simulink model "robot_circular"  (Simulink 8.2)
settings: Solver=FixedStepDiscrete  StartTime=0.0  StopTime=100  FixedStep=0.1  RelTol=1e-3
values from neighbouring files (symbols this model uses):
  Link1 = [pi/2, 0, pi/2, 0]    [robot_parameters.m]
  Link2 = [0, 0.404, pi/2, 0]    [robot_parameters.m]
  Link3 = [-pi/2, 0, 0, 0]    [robot_parameters.m]
  Link4 = [pi/2, 0.025, 0, 0.405]    [robot_parameters.m]
  Link5 = [pi/2, 0, pi/2, 0]    [robot_parameters.m]
  Link6 = [0, 0, pi/2, 0]    [robot_parameters.m]
  NoOfLinks = 6    [robot_parameters.m]
libraries: vrlib x3, instrumentlib x2, dspnetwork x2, simulink x2, utility x1
settings Model: Creator=angelosanto  LastModifiedBy=shashank  BufferReuse=off
settings DataIOCC: ReturnWorkspaceOutputs=on
settings OptimizationCC: BlockReduction=off  BooleanDataType=off  ConditionallyExecuteInputs=off  InlineParams=on  OptimizeBlockIOStorage=off  BufferReuse=off  ExpressionFolding=off  LocalBlockOutputs=off
settings RTWCC: GenCodeOnly=on  GenerateMakefile=off

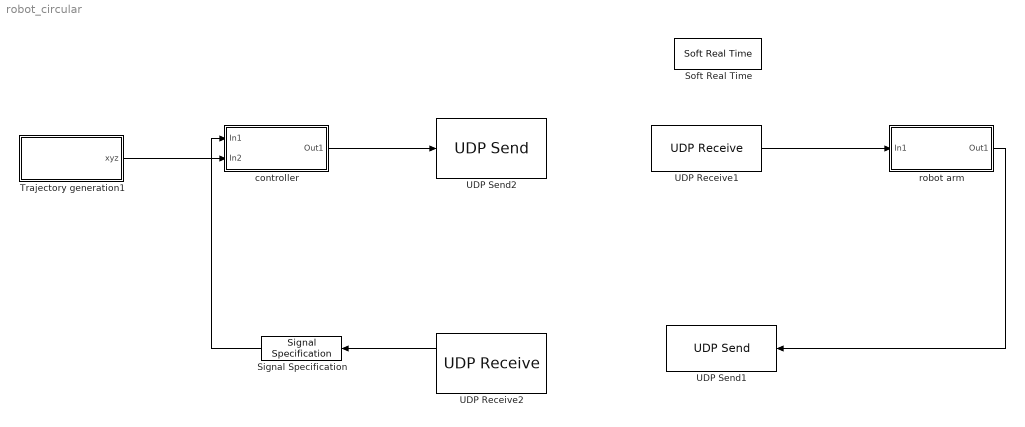
== system robot_circular ==
  Signal Specification : SignalSpecification  OutMin=6  OutMax=6  OutDataTypeStr=double
      settings: LockScale=on
  Soft Real Time : utility/Soft Real Time  x=0.5
  Trajectory generation1 : Subsystem
  UDP Receive1 : instrumentlib/UDP Receive  Priority=3  Host=localhost  Port=9090  LocalPort=9090  DataSize="[6  1]"  EnableBlockingMode=on  Timeout=10  SampleTime=0.1  DataType=double  ByteOrder=BigEndian
  UDP Receive2 : dspnetwork/UDP Receive  localURL='0.0.0.0'  localPort=9093  remoteURL='0.0.0.0'  remotePort=-1  recvBufferSize=8192  dims=6  signalDatatype=double  isVarSize=off  showBlockingTime=on  blockingTime=inf  sampletime=0.1  blockPlatform=LINUX
  UDP Send1 : instrumentlib/UDP Send  Priority=5  Host=localhost  Port=9092  LocalPort=9092  EnableBlockingMode=on  ByteOrder=BigEndian
  UDP Send2 : dspnetwork/UDP Send  remoteURL='localhost'  remotePort=9090  localURL='0.0.0.0'  localPortSource=Specify via dialog  localPort=9091  sampletime=-1  blockPlatform=LINUX  separateLengthPort=0
  controller : Subsystem
  robot arm : Subsystem  Priority=4
  wires:
  UDP Receive1/1 -> robot arm/1(In1)
  robot arm/1(Out1) -> UDP Send1/1
  controller/1(Out1) -> UDP Send2/1
  Trajectory generation1/1(xyz) -> controller/2(In2)
  UDP Receive2/1 -> Signal Specification/1
  Signal Specification/1 -> controller/1(In1)

== system robot_circular/Trajectory generation1 ==
  Bus Creator : BusCreator  Inputs='x','y','z'
  Constant1 : Constant  Value=0
  Constant4 : Constant
  Display : Display
  Fcn : Fcn  Expr=0.1*cos(u)+0.5
  Fcn1 : Fcn  Expr=0.1*sin(u)
  Fcn2 : Fcn  Expr=u/30
  Memory1 : Memory
  Sum1 : Sum  Inputs=|++
  xyz : Outport
  wires:
  Constant4/1 -> Sum1/2
  Sum1/1 -> Memory1/1, Display/1, Fcn2/1
  Memory1/1 -> Sum1/1
  Bus Creator/1 -> xyz/1
  Fcn1/1 -> Bus Creator/2  "y"
  Fcn/1 -> Bus Creator/1  "x"
  Fcn2/1 -> Fcn1/1, Fcn/1
  Constant1/1 -> Bus Creator/3  "z"

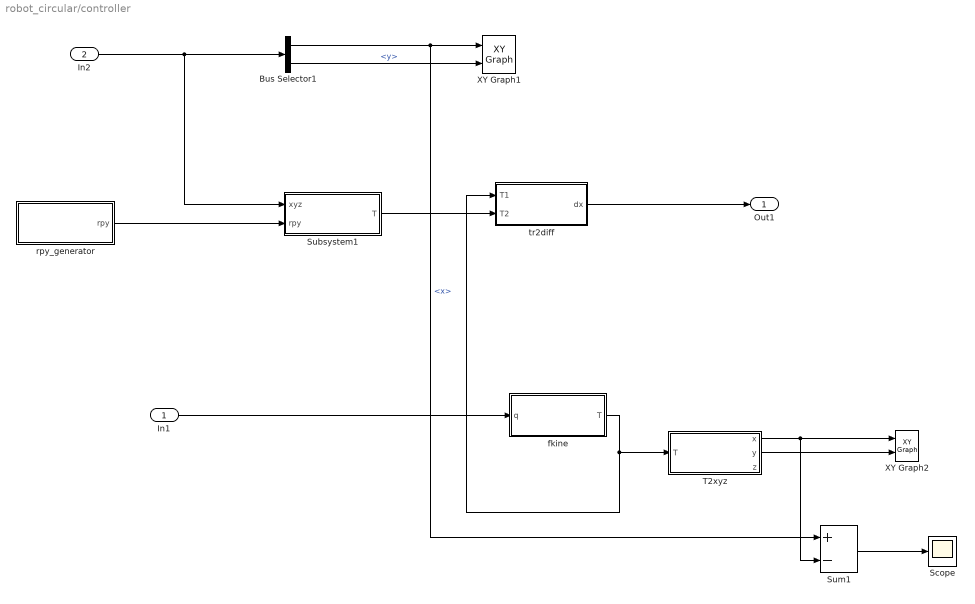
== system robot_circular/controller ==
  In1 : Inport
  In2 : Inport  Port=2
  Bus Selector1 : BusSelector  OutputSignals=x,y
  Scope : Scope
      settings: YMin=-0.03  YMax=-0.01
  Subsystem1 : Subsystem
  Sum1 : Sum  Inputs=+-
  T2xyz : Subsystem
  XY Graph1 : simulink/Sinks/XY Graph  xmin=-0.2  xmax=0.8  ymin=-0.5  ymax=0.5  st=-1
  XY Graph2 : simulink/Sinks/XY Graph  xmin=-0.2  xmax=0.8  ymin=-0.5  ymax=0.5  st=-1
  fkine : Subsystem  TreatAsAtomicUnit=on
  rpy_generator : Subsystem
  tr2diff : Subsystem
  Out1 : Outport
  wires:
  T2xyz/1(x) -> Sum1/2, XY Graph2/1
  fkine/1(T) -> tr2diff/1(T1), T2xyz/1(T)
  rpy_generator/1(rpy) -> Subsystem1/2(rpy)
  Bus Selector1/1 -> Sum1/1, XY Graph1/1  "<x>"
  Subsystem1/1(T) -> tr2diff/2(T2)
  Sum1/1 -> Scope/1
  Bus Selector1/2 -> XY Graph1/2  "<y>"
  T2xyz/2(y) -> XY Graph2/2
  In2/1 -> Subsystem1/1(xyz), Bus Selector1/1
  tr2diff/1(dx) -> Out1/1
  In1/1 -> fkine/1(q)

== system robot_circular/robot arm ==
  In1 : Inport
  Delay : Memory  X0=[pi/2; pi/2; 0; 0; pi/2; pi/2]  InheritSampleTime=on
  Gain1 : Gain  Gain=0.1
  Product : Product  Multiplication=Matrix(*)  RndMeth=Zero
  Scope5 : Scope
      settings: YMin=-0.02  YMax=0.0175  SaveName=ScopeData2
  Sum : Sum
  ijacob : Product  Inputs=/  Multiplication=Matrix(*)  RndMeth=Zero
  jacobn : Subsystem  TreatAsAtomicUnit=on
  Out1 : Outport
  wires:
  jacobn/1(Out1) -> ijacob/1
  ijacob/1 -> Product/1
  Sum/1 -> Delay/1
  Delay/1 -> Out1/1, jacobn/1(q), Sum/2
  Product/1 -> Gain1/1
  Gain1/1 -> Scope5/1, Sum/1
  In1/1 -> Product/2

== system robot_circular/controller/Subsystem1 ==
  xyz : Inport
  rpy : Inport  Port=2
  Bus Selector : BusSelector  OutputSignals=x,y,z
  Bus Selector1 : BusSelector  OutputSignals=roll,pitch,yaw
  Product : Product  Multiplication=Matrix(*)  RndMeth=Zero
  rpy2T : Subsystem
  xyz2T : Subsystem
  T : Outport
  wires:
  xyz/1 -> Bus Selector/1
  Bus Selector/1 -> xyz2T/1(x)  "<x>"
  Bus Selector/2 -> xyz2T/2(y)  "<y>"
  Bus Selector/3 -> xyz2T/3(z)  "<z>"
  xyz2T/1(T) -> Product/1
  Product/1 -> T/1
  rpy2T/1(T) -> Product/2
  rpy/1 -> Bus Selector1/1
  Bus Selector1/1 -> rpy2T/1(roll)  "<roll>"
  Bus Selector1/2 -> rpy2T/2(pitch)  "<pitch>"
  Bus Selector1/3 -> rpy2T/3(yaw)  "<yaw>"

== system robot_circular/controller/T2xyz ==
  T : Inport
  Selector : Selector  NumberOfDimensions=2  InputPortWidth=3  IndexOptions=Index vector (dialog),Index vector (dialog)  Indices=1,4  OutputSizes=1,1
  Selector1 : Selector  NumberOfDimensions=2  InputPortWidth=3  IndexOptions=Index vector (dialog),Index vector (dialog)  Indices=2,4  OutputSizes=1,1
  Selector2 : Selector  NumberOfDimensions=2  InputPortWidth=3  IndexOptions=Index vector (dialog),Index vector (dialog)  Indices=3,4  OutputSizes=1,1
  x : Outport
  y : Outport  Port=2
  z : Outport  Port=3
  wires:
  Selector/1 -> x/1
  Selector1/1 -> y/1
  Selector2/1 -> z/1
  T/1 -> Selector/1, Selector2/1, Selector1/1

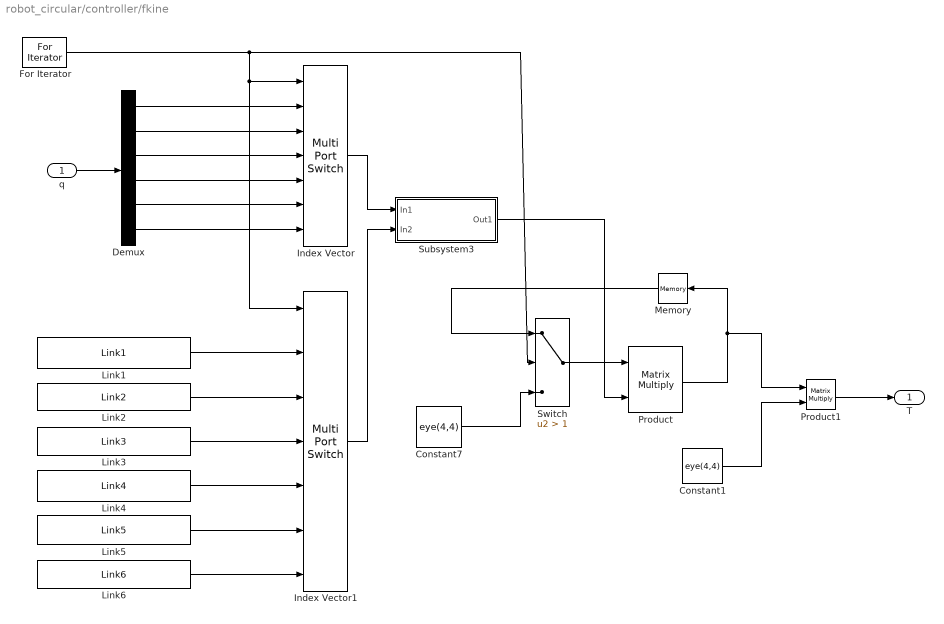
== system robot_circular/controller/fkine ==
  q : Inport
  Constant1 : Constant  Value=eye(4,4)
  Constant7 : Constant  Value=eye(4,4)
  Demux : Demux  Outputs=6
  For Iterator : ForIterator  IterationLimit=NoOfLinks
  Index Vector : MultiPortSwitch  Inputs=6
  Index Vector1 : MultiPortSwitch  Inputs=6
  Link1 : Constant  Value=Link1
  Link2 : Constant  Value=Link2
  Link3 : Constant  Value=Link3
  Link4 : Constant  Value=Link4
  Link5 : Constant  Value=Link5
  Link6 : Constant  Value=Link6
  Memory : Memory  X0=eye(4,4)  InheritSampleTime=on
  Product : Product  Multiplication=Matrix(*)  RndMeth=Zero
  Product1 : Product  Multiplication=Matrix(*)  RndMeth=Zero
  Subsystem3 : Subsystem
  Switch : Switch  Criteria=u2 > Threshold  Threshold=1
  T : Outport
  wires:
  Memory/1 -> Switch/1
  Switch/1 -> Product/1
  Subsystem3/1(Out1) -> Product/2
  Constant7/1 -> Switch/3
  Product/1 -> Product1/1, Memory/1
  Index Vector1/1 -> Subsystem3/2(In2)
  Index Vector/1 -> Subsystem3/1(In1)
  Demux/6 -> Index Vector/7
  Demux/5 -> Index Vector/6
  Demux/4 -> Index Vector/5
  Demux/3 -> Index Vector/4
  Demux/2 -> Index Vector/3
  Demux/1 -> Index Vector/2
  q/1 -> Demux/1
  Link6/1 -> Index Vector1/7
  Link5/1 -> Index Vector1/6
  Link4/1 -> Index Vector1/5
  Link3/1 -> Index Vector1/4
  Link2/1 -> Index Vector1/3
  Link1/1 -> Index Vector1/2
  For Iterator/1 -> Switch/2, Index Vector1/1, Index Vector/1
  Product1/1 -> T/1
  Constant1/1 -> Product1/2

== system robot_circular/controller/rpy_generator ==
  Bus Creator1 : BusCreator  Inputs=3
  Constant : Constant  Value=0  VectorParams1D=off
  Constant2 : Constant  Value=0
  Constant3 : Constant  Value=0
  rpy : Outport
  wires:
  Constant2/1 -> Bus Creator1/2  "pitch"
  Constant/1 -> Bus Creator1/1  "roll"
  Constant3/1 -> Bus Creator1/3  "yaw"
  Bus Creator1/1 -> rpy/1

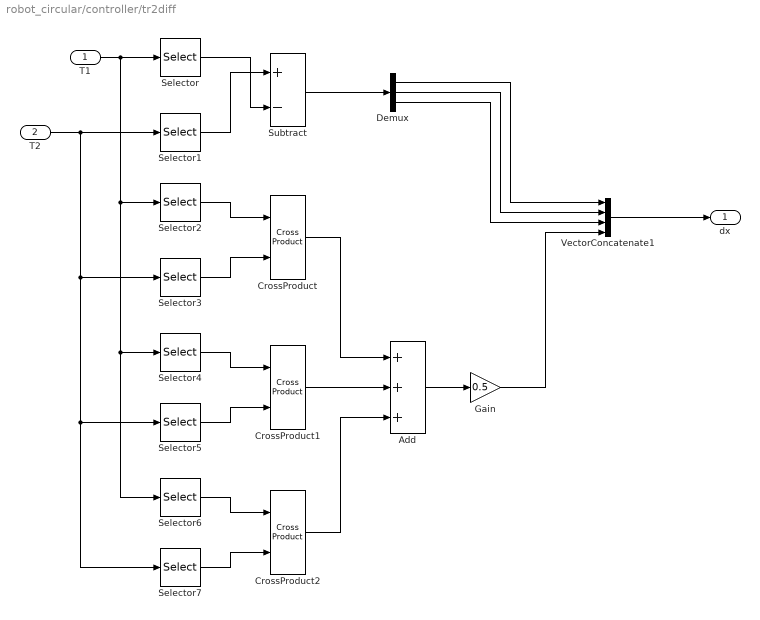
== system robot_circular/controller/tr2diff ==
  T1 : Inport
  T2 : Inport  Port=2
  Add : Sum  Inputs=+++
  CrossProduct : vrlib/Utilities/Cross Product
  CrossProduct1 : vrlib/Utilities/Cross Product
  CrossProduct2 : vrlib/Utilities/Cross Product
  Demux : Demux  Outputs=3
  Gain : Gain  Gain=0.5
  Selector : Selector  NumberOfDimensions=2  InputPortWidth=3  IndexOptions=Index vector (dialog),Index vector (dialog)  Indices=[1:3],4  OutputSizes=1,1
  Selector1 : Selector  NumberOfDimensions=2  InputPortWidth=3  IndexOptions=Index vector (dialog),Index vector (dialog)  Indices=[1:3],4  OutputSizes=1,1
  Selector2 : Selector  NumberOfDimensions=2  InputPortWidth=3  IndexOptions=Index vector (dialog),Index vector (dialog)  Indices=[1:3],1  OutputSizes=1,1
  Selector3 : Selector  NumberOfDimensions=2  InputPortWidth=3  IndexOptions=Index vector (dialog),Index vector (dialog)  Indices=[1:3],1  OutputSizes=1,1
  Selector4 : Selector  NumberOfDimensions=2  InputPortWidth=3  IndexOptions=Index vector (dialog),Index vector (dialog)  Indices=[1:3],2  OutputSizes=1,1
  Selector5 : Selector  NumberOfDimensions=2  InputPortWidth=3  IndexOptions=Index vector (dialog),Index vector (dialog)  Indices=[1:3],2  OutputSizes=1,1
  Selector6 : Selector  NumberOfDimensions=2  InputPortWidth=3  IndexOptions=Index vector (dialog),Index vector (dialog)  Indices=[1:3],3  OutputSizes=1,1
  Selector7 : Selector  NumberOfDimensions=2  InputPortWidth=3  IndexOptions=Index vector (dialog),Index vector (dialog)  Indices=[1:3],3  OutputSizes=1,1
  Subtract : Sum  Inputs=+-
  VectorConcatenate1 : Concatenate  NumInputs=4
  dx : Outport
  wires:
  T1/1 -> Selector/1, Selector2/1, Selector6/1, Selector4/1
  T2/1 -> Selector1/1, Selector7/1, Selector5/1, Selector3/1
  Selector1/1 -> Subtract/1
  Selector/1 -> Subtract/2
  Selector2/1 -> CrossProduct/1
  Selector3/1 -> CrossProduct/2
  Selector4/1 -> CrossProduct1/1
  Selector5/1 -> CrossProduct1/2
  Selector6/1 -> CrossProduct2/1
  Selector7/1 -> CrossProduct2/2
  CrossProduct/1 -> Add/1
  CrossProduct1/1 -> Add/2
  CrossProduct2/1 -> Add/3
  Add/1 -> Gain/1
  VectorConcatenate1/1 -> dx/1
  Subtract/1 -> Demux/1
  Demux/1 -> VectorConcatenate1/1
  Demux/2 -> VectorConcatenate1/2
  Demux/3 -> VectorConcatenate1/3
  Gain/1 -> VectorConcatenate1/4

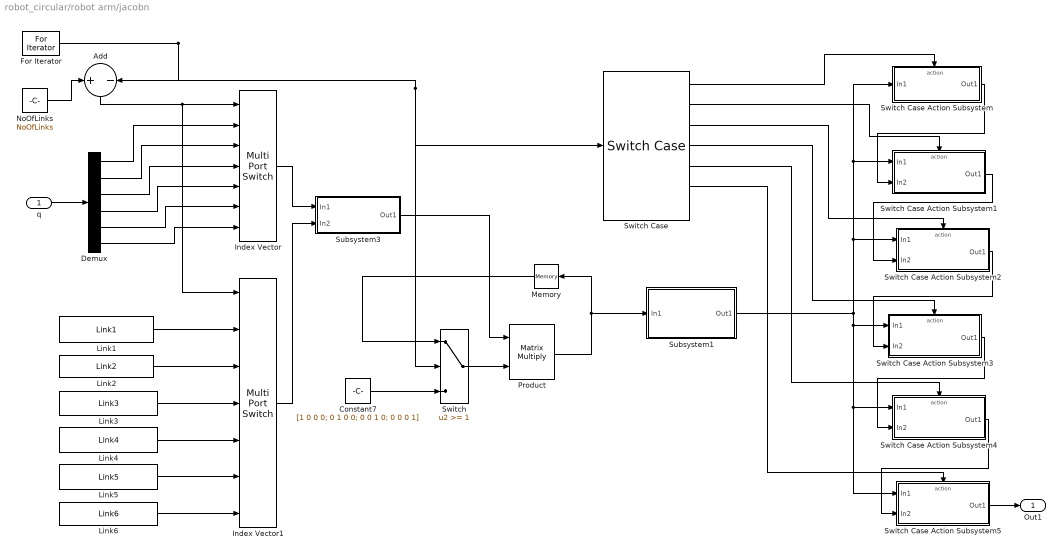
== system robot_circular/robot arm/jacobn ==
  q : Inport
  Add : Sum  Inputs=+-
  Constant7 : Constant  Value=[1 0 0 0; 0 1 0 0; 0 0 1 0; 0 0 0 1]
  Demux : Demux  Outputs=6
  For Iterator : ForIterator  IterationLimit=NoOfLinks
  Index Vector : MultiPortSwitch  DataPortOrder=Zero-based contiguous  Inputs=6  zeroidx=on
  Index Vector1 : MultiPortSwitch  DataPortOrder=Zero-based contiguous  Inputs=6  zeroidx=on
  Link1 : Constant  Value=Link1
  Link2 : Constant  Value=Link2
  Link3 : Constant  Value=Link3
  Link4 : Constant  Value=Link4
  Link5 : Constant  Value=Link5
  Link6 : Constant  Value=Link6
  Memory : Memory  X0=[1 0 0 0; 0 1 0 0; 0 0 1 0; 0 0 0 1]  InheritSampleTime=on
  NoOfLinks : Constant  Value=NoOfLinks
  Product : Product  Multiplication=Matrix(*)  RndMeth=Zero
  Subsystem1 : Subsystem
  Subsystem3 : Subsystem
  Switch : Switch  Threshold=1
  Switch Case : SwitchCase  CaseConditions={1, 2, 3, 4, 5, 6}
  Switch Case Action Subsystem : Subsystem  TreatAsAtomicUnit=on
  Switch Case Action Subsystem1 : Subsystem  TreatAsAtomicUnit=on
  Switch Case Action Subsystem2 : Subsystem  TreatAsAtomicUnit=on
  Switch Case Action Subsystem3 : Subsystem  TreatAsAtomicUnit=on
  Switch Case Action Subsystem4 : Subsystem  TreatAsAtomicUnit=on
  Switch Case Action Subsystem5 : Subsystem  TreatAsAtomicUnit=on
  Out1 : Outport
  wires:
  NoOfLinks/1 -> Add/1
  For Iterator/1 -> Add/2, Switch/2, Switch Case/1
  Add/1 -> Index Vector/1, Index Vector1/1
  Link1/1 -> Index Vector1/2
  Link2/1 -> Index Vector1/3
  Link3/1 -> Index Vector1/4
  Link4/1 -> Index Vector1/5
  Link5/1 -> Index Vector1/6
  Link6/1 -> Index Vector1/7
  q/1 -> Demux/1
  Demux/1 -> Index Vector/2
  Demux/2 -> Index Vector/3
  Demux/3 -> Index Vector/4
  Demux/4 -> Index Vector/5
  Demux/5 -> Index Vector/6
  Demux/6 -> Index Vector/7
  Index Vector/1 -> Subsystem3/1(In1)
  Index Vector1/1 -> Subsystem3/2(In2)
  Product/1 -> Memory/1, Subsystem1/1(In1)
  Constant7/1 -> Switch/3
  Subsystem3/1(Out1) -> Product/1
  Switch/1 -> Product/2
  Memory/1 -> Switch/1
  Subsystem1/1(Out1) -> Switch Case Action Subsystem/1(In1), Switch Case Action Subsystem1/1(In1), Switch Case Action Subsystem2/1(In1), Switch Case Action Subsystem5/1(In1), Switch Case Action Subsystem4/1(In1), Switch Case Action Subsystem3/1(In1)
  Switch Case/1 -> Switch Case Action Subsystem/Action
  Switch Case/2 -> Switch Case Action Subsystem1/Action
  Switch Case/3 -> Switch Case Action Subsystem2/Action
  Switch Case/4 -> Switch Case Action Subsystem3/Action
  Switch Case/5 -> Switch Case Action Subsystem4/Action
  Switch Case/6 -> Switch Case Action Subsystem5/Action
  Switch Case Action Subsystem5/1(Out1) -> Out1/1
  Switch Case Action Subsystem1/1(Out1) -> Switch Case Action Subsystem2/2(In2)
  Switch Case Action Subsystem/1(Out1) -> Switch Case Action Subsystem1/2(In2)
  Switch Case Action Subsystem2/1(Out1) -> Switch Case Action Subsystem3/2(In2)
  Switch Case Action Subsystem3/1(Out1) -> Switch Case Action Subsystem4/2(In2)
  Switch Case Action Subsystem4/1(Out1) -> Switch Case Action Subsystem5/2(In2)

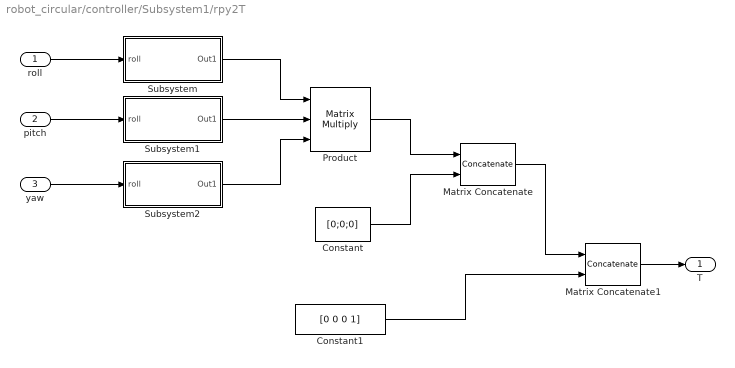
== system robot_circular/controller/Subsystem1/rpy2T ==
  roll : Inport
  pitch : Inport  Port=2
  yaw : Inport  Port=3
  Constant : Constant  Value=[0;0;0]
  Constant1 : Constant  Value=[0 0 0 1]  VectorParams1D=off
  Matrix Concatenate : Concatenate  Mode=Multidimensional array  ConcatenateDimension=2
  Matrix Concatenate1 : Concatenate  Mode=Multidimensional array
  Product : Product  Inputs=3  Multiplication=Matrix(*)  RndMeth=Zero
  Subsystem : Subsystem
  Subsystem1 : Subsystem
  Subsystem2 : Subsystem
  T : Outport
  wires:
  roll/1 -> Subsystem/1(roll)
  pitch/1 -> Subsystem1/1(roll)
  yaw/1 -> Subsystem2/1(roll)
  Subsystem/1(Out1) -> Product/1
  Subsystem1/1(Out1) -> Product/2
  Subsystem2/1(Out1) -> Product/3
  Product/1 -> Matrix Concatenate/1
  Constant/1 -> Matrix Concatenate/2
  Matrix Concatenate/1 -> Matrix Concatenate1/1
  Constant1/1 -> Matrix Concatenate1/2
  Matrix Concatenate1/1 -> T/1

== system robot_circular/controller/Subsystem1/xyz2T ==
  x : Inport
  y : Inport  Port=2
  z : Inport  Port=3
  Constant : Constant  Value=eye(3)
  Constant1 : Constant  Value=[0 0 0 1]  VectorParams1D=off
  Matrix Concatenate : Concatenate  Mode=Multidimensional array  ConcatenateDimension=2
  Matrix Concatenate1 : Concatenate  Mode=Multidimensional array
  Vector Concatenate : Concatenate  NumInputs=3
  T : Outport
  wires:
  x/1 -> Vector Concatenate/1
  y/1 -> Vector Concatenate/2
  z/1 -> Vector Concatenate/3
  Constant/1 -> Matrix Concatenate/1
  Vector Concatenate/1 -> Matrix Concatenate/2
  Matrix Concatenate/1 -> Matrix Concatenate1/1
  Constant1/1 -> Matrix Concatenate1/2
  Matrix Concatenate1/1 -> T/1

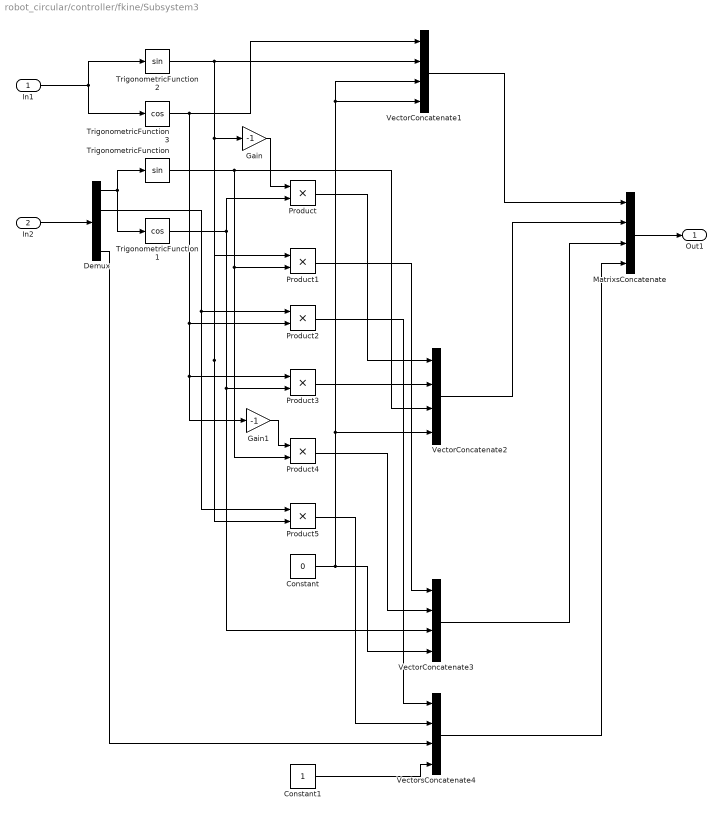
== system robot_circular/controller/fkine/Subsystem3 ==
  In1 : Inport
  In2 : Inport  Port=2
  Constant : Constant  Value=0
  Constant1 : Constant
  Demux : Demux
  Gain : Gain  Gain=-1
  Gain1 : Gain  Gain=-1
  MatrixsConcatenate : Concatenate  NumInputs=4  Mode=Multidimensional array  ConcatenateDimension=2
  Product{,1..5} (6 alike) : Product  RndMeth=Zero
  TrigonometricFunction : Trigonometry
  TrigonometricFunction1 : Trigonometry  Operator=cos
  TrigonometricFunction2 : Trigonometry
  TrigonometricFunction3 : Trigonometry  Operator=cos
  VectorConcatenate1 : Concatenate  NumInputs=4  ConcatenateDimension=2
  VectorConcatenate2 : Concatenate  NumInputs=4  ConcatenateDimension=2
  VectorConcatenate3 : Concatenate  NumInputs=4  ConcatenateDimension=2
  VectorsConcatenate4 : Concatenate  NumInputs=4  ConcatenateDimension=2
  Out1 : Outport
  wires:
  VectorsConcatenate4/1 -> MatrixsConcatenate/4
  VectorConcatenate3/1 -> MatrixsConcatenate/3
  VectorConcatenate2/1 -> MatrixsConcatenate/2
  VectorConcatenate1/1 -> MatrixsConcatenate/1
  MatrixsConcatenate/1 -> Out1/1
  Constant1/1 -> VectorsConcatenate4/4
  Constant/1 -> VectorConcatenate1/3, VectorConcatenate1/4, VectorConcatenate2/4, VectorConcatenate3/4
  Gain1/1 -> Product4/1
  Product3/1 -> VectorConcatenate2/2
  Demux/2 -> Product5/1, Product2/1
  TrigonometricFunction/1 -> Product1/2, Product4/2, VectorConcatenate2/3
  TrigonometricFunction3/1 -> VectorConcatenate1/1, Gain1/1, Product3/1, Product2/2
  TrigonometricFunction1/1 -> VectorConcatenate3/3, Product3/2, Product/2
  Gain/1 -> Product/1
  TrigonometricFunction2/1 -> Product1/1, Product5/2, Gain/1, VectorConcatenate1/2
  Demux/1 -> TrigonometricFunction1/1, TrigonometricFunction/1
  In1/1 -> TrigonometricFunction3/1, TrigonometricFunction2/1
  In2/1 -> Demux/1
  Product/1 -> VectorConcatenate2/1
  Product4/1 -> VectorConcatenate3/2
  Product1/1 -> VectorConcatenate3/1
  Product2/1 -> VectorsConcatenate4/1
  Product5/1 -> VectorsConcatenate4/2
  Demux/4 -> VectorsConcatenate4/3

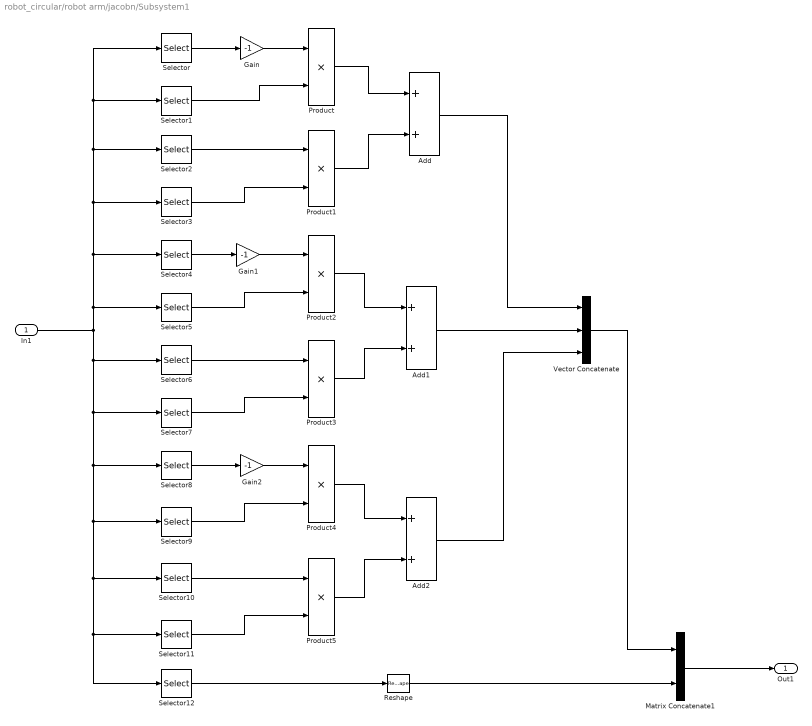
== system robot_circular/robot arm/jacobn/Subsystem1 ==
  In1 : Inport
  Add : Sum
  Add1 : Sum
  Add2 : Sum
  Gain : Gain  Gain=-1
  Gain1 : Gain  Gain=-1
  Gain2 : Gain  Gain=-1
  Matrix Concatenate1 : Concatenate  Mode=Multidimensional array
  Product{,1..5} (6 alike) : Product  RndMeth=Zero
  Reshape : Reshape  OutputDimensionality=Customize  OutputDimensions=[3,1]
  Selector : Selector  NumberOfDimensions=2  InputPortWidth=3  IndexOptions=Index vector (dialog),Index vector (dialog)  Indices=1,1  OutputSizes=1,1
  Selector1 : Selector  NumberOfDimensions=2  InputPortWidth=3  IndexOptions=Index vector (dialog),Index vector (dialog)  Indices=2,4  OutputSizes=1,1
  Selector10 : Selector  NumberOfDimensions=2  InputPortWidth=3  IndexOptions=Index vector (dialog),Index vector (dialog)  Indices=2,3  OutputSizes=1,1
  Selector11 : Selector  NumberOfDimensions=2  InputPortWidth=3  IndexOptions=Index vector (dialog),Index vector (dialog)  Indices=1,4  OutputSizes=1,1
  Selector12 : Selector  NumberOfDimensions=2  InputPortWidth=3  IndexOptions=Index vector (dialog),Index vector (dialog)  Indices=3,[1:3]  OutputSizes=1,1
  Selector2 : Selector  NumberOfDimensions=2  InputPortWidth=3  IndexOptions=Index vector (dialog),Index vector (dialog)  Indices=2,1  OutputSizes=1,1
  Selector3 : Selector  NumberOfDimensions=2  InputPortWidth=3  IndexOptions=Index vector (dialog),Index vector (dialog)  Indices=1,4  OutputSizes=1,1
  Selector4 : Selector  NumberOfDimensions=2  InputPortWidth=3  IndexOptions=Index vector (dialog),Index vector (dialog)  Indices=1,2  OutputSizes=1,1
  Selector5 : Selector  NumberOfDimensions=2  InputPortWidth=3  IndexOptions=Index vector (dialog),Index vector (dialog)  Indices=2,4  OutputSizes=1,1
  Selector6 : Selector  NumberOfDimensions=2  InputPortWidth=3  IndexOptions=Index vector (dialog),Index vector (dialog)  Indices=2,2  OutputSizes=1,1
  Selector7 : Selector  NumberOfDimensions=2  InputPortWidth=3  IndexOptions=Index vector (dialog),Index vector (dialog)  Indices=1,4  OutputSizes=1,1
  Selector8 : Selector  NumberOfDimensions=2  InputPortWidth=3  IndexOptions=Index vector (dialog),Index vector (dialog)  Indices=1,3  OutputSizes=1,1
  Selector9 : Selector  NumberOfDimensions=2  InputPortWidth=3  IndexOptions=Index vector (dialog),Index vector (dialog)  Indices=2,4  OutputSizes=1,1
  Vector Concatenate : Concatenate  NumInputs=3
  Out1 : Outport
  wires:
  Selector/1 -> Gain/1
  In1/1 -> Selector/1, Selector1/1, Selector2/1, Selector3/1, Selector4/1, Selector5/1, Selector10/1, Selector11/1, Selector12/1, Selector9/1, Selector8/1, Selector7/1, Selector6/1
  Gain/1 -> Product/1
  Selector1/1 -> Product/2
  Selector2/1 -> Product1/1
  Selector3/1 -> Product1/2
  Selector4/1 -> Gain1/1
  Gain1/1 -> Product2/1
  Selector5/1 -> Product2/2
  Selector6/1 -> Product3/1
  Selector7/1 -> Product3/2
  Selector8/1 -> Gain2/1
  Gain2/1 -> Product4/1
  Selector9/1 -> Product4/2
  Selector10/1 -> Product5/1
  Selector11/1 -> Product5/2
  Product/1 -> Add/1
  Product1/1 -> Add/2
  Product2/1 -> Add1/1
  Product3/1 -> Add1/2
  Product4/1 -> Add2/1
  Product5/1 -> Add2/2
  Add/1 -> Vector Concatenate/1
  Add1/1 -> Vector Concatenate/2
  Add2/1 -> Vector Concatenate/3
  Vector Concatenate/1 -> Matrix Concatenate1/1
  Selector12/1 -> Reshape/1
  Matrix Concatenate1/1 -> Out1/1
  Reshape/1 -> Matrix Concatenate1/2

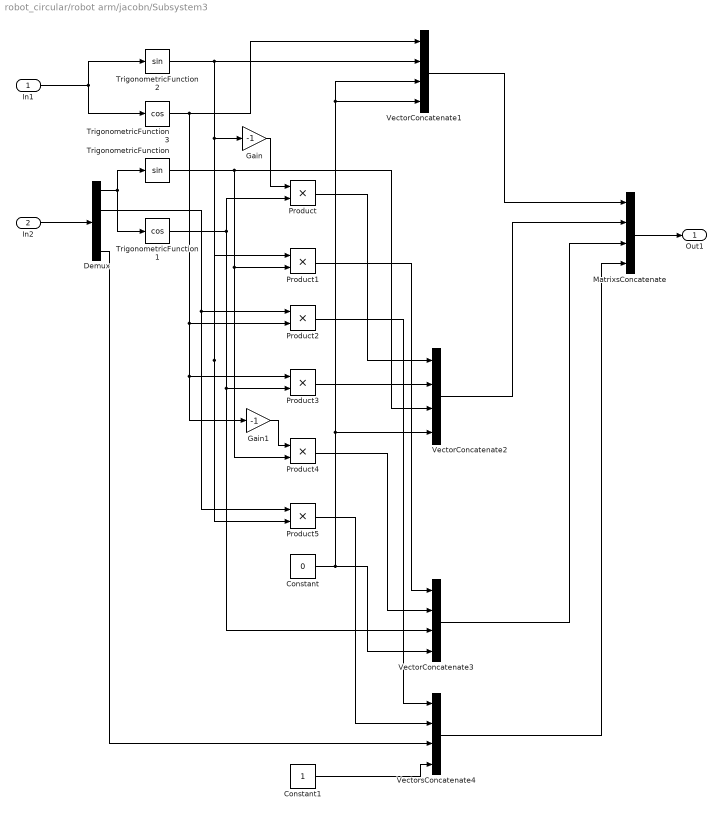
== system robot_circular/robot arm/jacobn/Subsystem3 ==
  In1 : Inport
  In2 : Inport  Port=2
  Constant : Constant  Value=0
  Constant1 : Constant
  Demux : Demux
  Gain : Gain  Gain=-1
  Gain1 : Gain  Gain=-1
  MatrixsConcatenate : Concatenate  NumInputs=4  Mode=Multidimensional array  ConcatenateDimension=2
  Product{,1..5} (6 alike) : Product  RndMeth=Zero
  TrigonometricFunction : Trigonometry
  TrigonometricFunction1 : Trigonometry  Operator=cos
  TrigonometricFunction2 : Trigonometry
  TrigonometricFunction3 : Trigonometry  Operator=cos
  VectorConcatenate1 : Concatenate  NumInputs=4  ConcatenateDimension=2
  VectorConcatenate2 : Concatenate  NumInputs=4  ConcatenateDimension=2
  VectorConcatenate3 : Concatenate  NumInputs=4  ConcatenateDimension=2
  VectorsConcatenate4 : Concatenate  NumInputs=4  ConcatenateDimension=2
  Out1 : Outport
  wires:
  VectorsConcatenate4/1 -> MatrixsConcatenate/4
  VectorConcatenate3/1 -> MatrixsConcatenate/3
  VectorConcatenate2/1 -> MatrixsConcatenate/2
  VectorConcatenate1/1 -> MatrixsConcatenate/1
  MatrixsConcatenate/1 -> Out1/1
  Constant1/1 -> VectorsConcatenate4/4
  Constant/1 -> VectorConcatenate1/3, VectorConcatenate1/4, VectorConcatenate2/4, VectorConcatenate3/4
  Gain1/1 -> Product4/1
  Product3/1 -> VectorConcatenate2/2
  Demux/2 -> Product5/1, Product2/1
  TrigonometricFunction/1 -> Product1/2, Product4/2, VectorConcatenate2/3
  TrigonometricFunction3/1 -> VectorConcatenate1/1, Gain1/1, Product3/1, Product2/2
  TrigonometricFunction1/1 -> VectorConcatenate3/3, Product3/2, Product/2
  Gain/1 -> Product/1
  TrigonometricFunction2/1 -> Product1/1, Product5/2, Gain/1, VectorConcatenate1/2
  Demux/1 -> TrigonometricFunction1/1, TrigonometricFunction/1
  In1/1 -> TrigonometricFunction3/1, TrigonometricFunction2/1
  In2/1 -> Demux/1
  Product/1 -> VectorConcatenate2/1
  Product4/1 -> VectorConcatenate3/2
  Product1/1 -> VectorConcatenate3/1
  Product2/1 -> VectorsConcatenate4/1
  Product5/1 -> VectorsConcatenate4/2
  Demux/4 -> VectorsConcatenate4/3

== system robot_circular/robot arm/jacobn/Switch Case Action Subsystem ==
  In1 : Inport
  Action Port : ActionPort  ActionType=case
  Matrix Concatenate : Concatenate  NumInputs=1  Mode=Multidimensional array  ConcatenateDimension=2
  Out1 : Outport
  wires:
  In1/1 -> Matrix Concatenate/1
  Matrix Concatenate/1 -> Out1/1

== system robot_circular/robot arm/jacobn/Switch Case Action Subsystem1 ==
  In1 : Inport
  In2 : Inport  Port=2
  Action Port : ActionPort  ActionType=case
  Matrix Concatenate : Concatenate  Mode=Multidimensional array  ConcatenateDimension=2
  Out1 : Outport
  wires:
  In1/1 -> Matrix Concatenate/1
  In2/1 -> Matrix Concatenate/2
  Matrix Concatenate/1 -> Out1/1

== system robot_circular/robot arm/jacobn/Switch Case Action Subsystem2 ==
  In1 : Inport
  In2 : Inport  Port=2
  Action Port : ActionPort  ActionType=case
  Matrix Concatenate : Concatenate  Mode=Multidimensional array  ConcatenateDimension=2
  Out1 : Outport
  wires:
  Matrix Concatenate/1 -> Out1/1
  In2/1 -> Matrix Concatenate/2
  In1/1 -> Matrix Concatenate/1

== system robot_circular/robot arm/jacobn/Switch Case Action Subsystem3 ==
  In1 : Inport
  In2 : Inport  Port=2
  Action Port : ActionPort  ActionType=case
  Matrix Concatenate : Concatenate  Mode=Multidimensional array  ConcatenateDimension=2
  Out1 : Outport
  wires:
  In1/1 -> Matrix Concatenate/1
  In2/1 -> Matrix Concatenate/2
  Matrix Concatenate/1 -> Out1/1

== system robot_circular/robot arm/jacobn/Switch Case Action Subsystem4 ==
  In1 : Inport
  In2 : Inport  Port=2
  Action Port : ActionPort  ActionType=case
  Matrix Concatenate : Concatenate  Mode=Multidimensional array  ConcatenateDimension=2
  Out1 : Outport
  wires:
  Matrix Concatenate/1 -> Out1/1
  In2/1 -> Matrix Concatenate/2
  In1/1 -> Matrix Concatenate/1

== system robot_circular/robot arm/jacobn/Switch Case Action Subsystem5 ==
  In1 : Inport
  In2 : Inport  Port=2
  Action Port : ActionPort  ActionType=case
  Matrix Concatenate : Concatenate  Mode=Multidimensional array  ConcatenateDimension=2
  Out1 : Outport
  wires:
  In1/1 -> Matrix Concatenate/1
  In2/1 -> Matrix Concatenate/2
  Matrix Concatenate/1 -> Out1/1

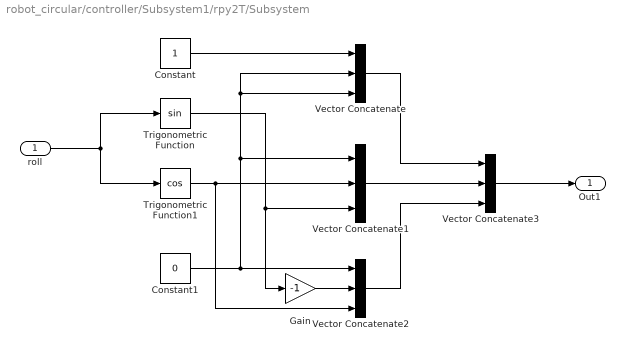
== system robot_circular/controller/Subsystem1/rpy2T/Subsystem ==
  roll : Inport
  Constant : Constant
  Constant1 : Constant  Value=0
  Gain : Gain  Gain=-1
  Trigonometric Function : Trigonometry
  Trigonometric Function1 : Trigonometry  Operator=cos
  Vector Concatenate : Concatenate  NumInputs=3
  Vector Concatenate1 : Concatenate  NumInputs=3
  Vector Concatenate2 : Concatenate  NumInputs=3
  Vector Concatenate3 : Concatenate  NumInputs=3  Mode=Multidimensional array  ConcatenateDimension=2
  Out1 : Outport
  wires:
  roll/1 -> Trigonometric Function/1, Trigonometric Function1/1
  Constant/1 -> Vector Concatenate/1
  Trigonometric Function1/1 -> Vector Concatenate1/2, Vector Concatenate2/3
  Trigonometric Function/1 -> Gain/1, Vector Concatenate1/3
  Vector Concatenate/1 -> Vector Concatenate3/1
  Vector Concatenate1/1 -> Vector Concatenate3/2
  Vector Concatenate2/1 -> Vector Concatenate3/3
  Constant1/1 -> Vector Concatenate/2, Vector Concatenate/3, Vector Concatenate1/1, Vector Concatenate2/1
  Gain/1 -> Vector Concatenate2/2
  Vector Concatenate3/1 -> Out1/1

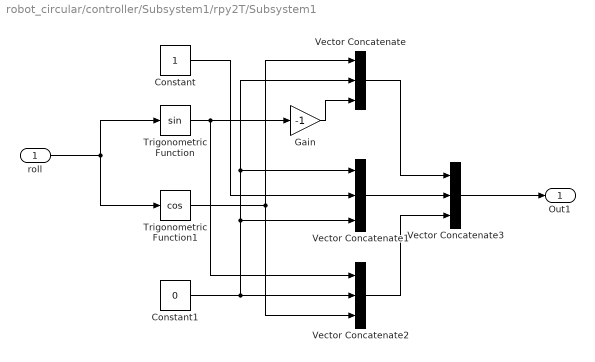
== system robot_circular/controller/Subsystem1/rpy2T/Subsystem1 ==
  roll : Inport
  Constant : Constant
  Constant1 : Constant  Value=0
  Gain : Gain  Gain=-1
  Trigonometric Function : Trigonometry
  Trigonometric Function1 : Trigonometry  Operator=cos
  Vector Concatenate : Concatenate  NumInputs=3
  Vector Concatenate1 : Concatenate  NumInputs=3
  Vector Concatenate2 : Concatenate  NumInputs=3
  Vector Concatenate3 : Concatenate  NumInputs=3  Mode=Multidimensional array  ConcatenateDimension=2
  Out1 : Outport
  wires:
  roll/1 -> Trigonometric Function/1, Trigonometric Function1/1
  Vector Concatenate/1 -> Vector Concatenate3/1
  Vector Concatenate1/1 -> Vector Concatenate3/2
  Vector Concatenate2/1 -> Vector Concatenate3/3
  Trigonometric Function1/1 -> Vector Concatenate/1, Vector Concatenate2/3
  Constant1/1 -> Vector Concatenate2/2, Vector Concatenate/2, Vector Concatenate1/1, Vector Concatenate1/3
  Trigonometric Function/1 -> Gain/1, Vector Concatenate2/1
  Constant/1 -> Vector Concatenate1/2
  Gain/1 -> Vector Concatenate/3
  Vector Concatenate3/1 -> Out1/1

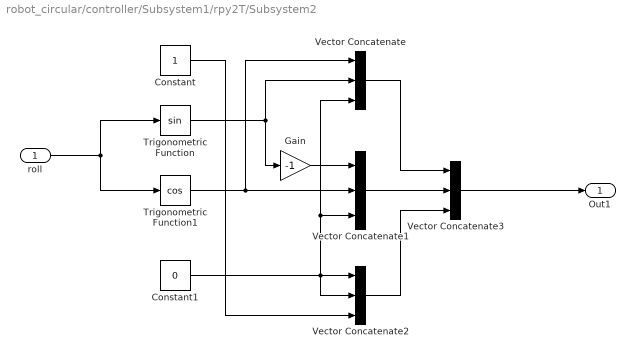
== system robot_circular/controller/Subsystem1/rpy2T/Subsystem2 ==
  roll : Inport
  Constant : Constant
  Constant1 : Constant  Value=0
  Gain : Gain  Gain=-1
  Trigonometric Function : Trigonometry
  Trigonometric Function1 : Trigonometry  Operator=cos
  Vector Concatenate : Concatenate  NumInputs=3
  Vector Concatenate1 : Concatenate  NumInputs=3
  Vector Concatenate2 : Concatenate  NumInputs=3
  Vector Concatenate3 : Concatenate  NumInputs=3  Mode=Multidimensional array  ConcatenateDimension=2
  Out1 : Outport
  wires:
  roll/1 -> Trigonometric Function/1, Trigonometric Function1/1
  Vector Concatenate/1 -> Vector Concatenate3/1
  Vector Concatenate1/1 -> Vector Concatenate3/2
  Vector Concatenate2/1 -> Vector Concatenate3/3
  Trigonometric Function1/1 -> Vector Concatenate/1, Vector Concatenate1/2
  Trigonometric Function/1 -> Vector Concatenate/2, Gain/1
  Constant1/1 -> Vector Concatenate/3, Vector Concatenate1/3, Vector Concatenate2/1, Vector Concatenate2/2
  Constant/1 -> Vector Concatenate2/3
  Gain/1 -> Vector Concatenate1/1
  Vector Concatenate3/1 -> Out1/1
